simulink model "control_sim_hw2_sim"  (R2023b)
settings: Solver=VariableStepAuto  StartTime=0.0  StopTime=10.0  RelTol=1e-3
settings Model: Creator=henry  LastModifiedBy=henry

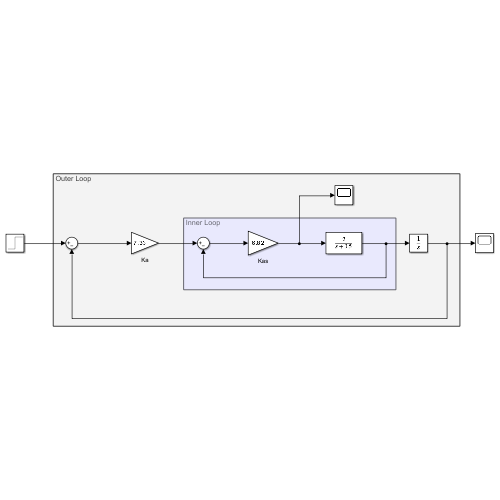
[thumbnail: Simulink's stored preview of the top-level diagram]
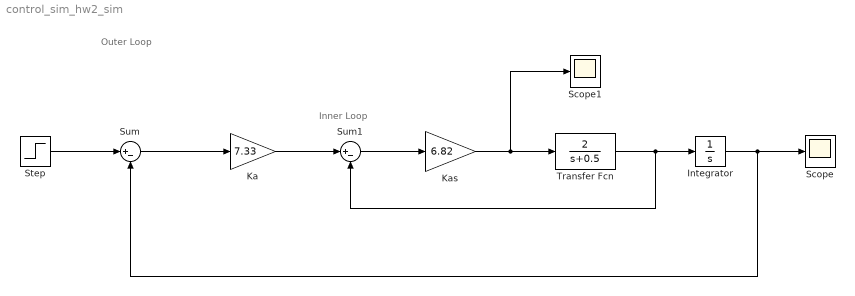
== system control_sim_hw2_sim ==
  note: Outer Loop
  note: Inner Loop
  Integrator : Integrator
  Ka : Gain  Gain=7.33
  Kas : Gain  Gain=6.82
  Scope : Scope
  Scope1 : Scope
  Step : Step  SampleTime=0
  Sum : Sum  Inputs=|+-
  Sum1 : Sum  Inputs=|+-
  Transfer Fcn : TransferFcn  Numerator=[2]  Denominator=[1 0.5]
  wires:
  Sum/1 -> Ka/1
  Ka/1 -> Sum1/1
  Sum1/1 -> Kas/1
  Kas/1 -> Scope1/1, Transfer Fcn/1
  Transfer Fcn/1 -> Sum1/2, Integrator/1
  Integrator/1 -> Sum/2, Scope/1
  Step/1 -> Sum/1
